simulink model "lab3"  (R2018a)
settings: Solver=FixedStepAuto  StartTime=0.0  StopTime=100  RelTol=1e-3  EnableMultiTasking=on
libraries: dspsnks4 x1, dspvision x1
settings Model: Creator=cvillal3  LastModifiedBy=cvillal3
settings CodeAppCC: StateflowObjectComments=on

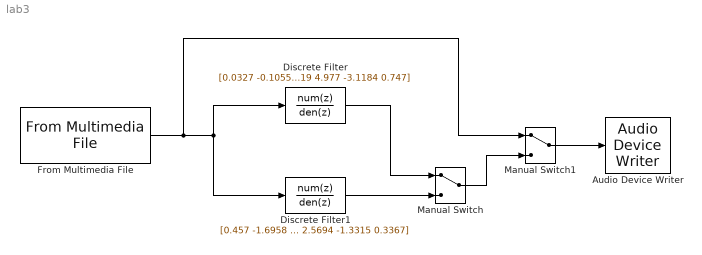
== system lab3 ==
  Audio Device Writer : dspsnks4/Audio Device Writer  Driver=DirectSound  Device=Default  InheritSampleRate=on  SampleRate=44100  BitDepth=16-bit integer  BufferSize=4096  NumBuffers=10  DefaultOutputChannelMapping=on  OutputChannelMapping=1:2  OutputNumUnderrunSamples=off  DriverIdx=1  DeviceWarnFlag=''
  Discrete Filter : DiscreteFilter  Numerator=[0.0327 -0.1055 0.1488 -0.1055 0.0327]  Denominator=[1 -3.6019 4.977 -3.1184 0.747]  InputProcessing=Columns as channels (frame based)
  Discrete Filter1 : DiscreteFilter  Numerator=[0.457 -1.6958 2.4838 -1.6958 0.457]  Denominator=[1 -2.3804 2.5694 -1.3315 0.3367]  InputProcessing=Columns as channels (frame based)
  From Multimedia File : dspvision/From Multimedia File  inputFilename=Kalimba.mp3  loop=on  numPlays=inf  outputStreams=Audio only  videoDataType=single  audioDataType=double  inheritSampleTime=on  userDefinedSampleTime=1/30  noAudioOutput=off  isIntensityVideo=off  fourcc=RGB  colorVideoFormat=Separate color signals  outputEOF=off  dataOrg=Column-major  audioFrameSize=1024  computeAudioFrameSize=off  outSamplingMode=Sample based
      settings: SourceProductBaseCode=VP
  Manual Switch : ManualSwitch
  Manual Switch1 : ManualSwitch
  wires:
  Discrete Filter1/1 -> Manual Switch/2
  Discrete Filter/1 -> Manual Switch/1
  Manual Switch/1 -> Manual Switch1/2
  From Multimedia File/1 -> Manual Switch1/1, Discrete Filter1/1, Discrete Filter/1
  Manual Switch1/1 -> Audio Device Writer/1
